simulink model "SSIV_Simulink_Com2"  (R2018a)
settings: Solver=FixedStepAuto  StartTime=0.0  StopTime=inf  FixedStep=.015  RelTol=1e-3  EnableMultiTasking=on
libraries: hdlsllib x51, raspberrypilib x16, simulink x10
(part 2 of 2)

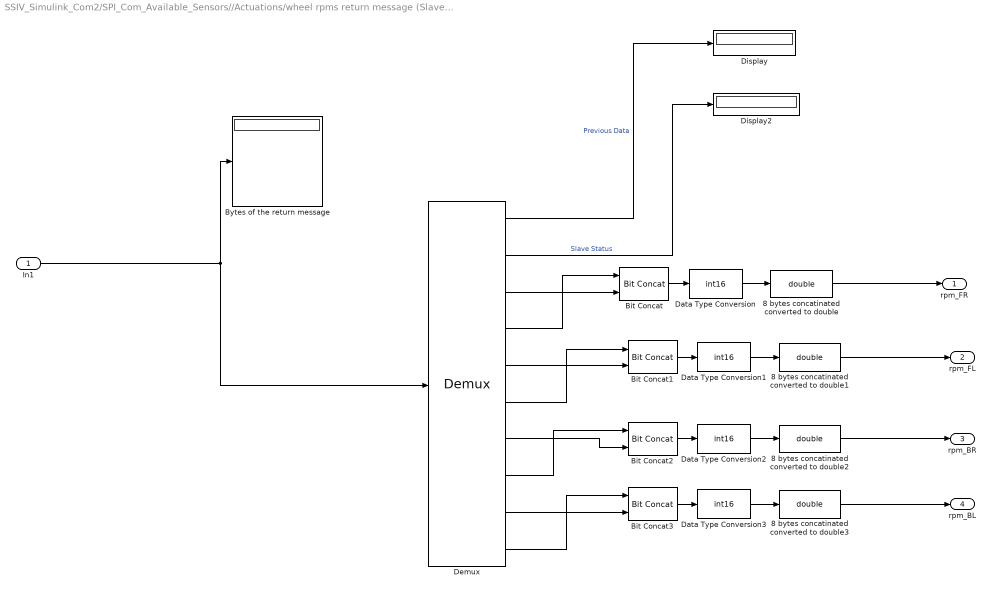
== system SSIV_Simulink_Com2/SPI_Com_Available_Sensors//Actuations/wheel rpms return message (Slave --> Master) ==
  In1 : Inport
  8 bytes concatinated converted to double{,1..3} (4 alike) : DataTypeConversion  OutDataTypeStr=double  RndMeth=Nearest
  Bit Concat{,1..3} (4 alike) : hdlsllib/Logic and Bit Operations/Bit Concat  numInputs=2
      settings: SourceProductName=HDL Coder  SourceProductBaseCode=HD
  Bytes of the return message : Display
      settings: Format=decimal (Stored Integer)
  Data Type Conversion{,1..3} (4 alike) : DataTypeConversion  OutDataTypeStr=int16  RndMeth=Nearest
  Demux : Demux  Outputs=10
  Display : Display
      settings: Format=binary (Stored Integer)
  Display2 : Display
      settings: Format=binary (Stored Integer)
  rpm_FR : Outport
  rpm_FL : Outport  Port=2
  rpm_BR : Outport  Port=3
  rpm_BL : Outport  Port=4
  wires:
  8 bytes concatinated converted to double/1 -> rpm_FR/1
  Demux/2 -> Display2/1  "Slave Status"
  Demux/1 -> Display/1  "Previous Data"
  In1/1 -> Bytes of the return message/1, Demux/1
  Bit Concat/1 -> Data Type Conversion/1
  Demux/4 -> Bit Concat/1
  Demux/3 -> Bit Concat/2
  Data Type Conversion/1 -> 8 bytes concatinated converted to double/1
  Data Type Conversion1/1 -> 8 bytes concatinated converted to double1/1
  Demux/5 -> Bit Concat1/2
  Demux/6 -> Bit Concat1/1
  Bit Concat1/1 -> Data Type Conversion1/1
  8 bytes concatinated converted to double1/1 -> rpm_FL/1
  8 bytes concatinated converted to double2/1 -> rpm_BR/1
  Bit Concat2/1 -> Data Type Conversion2/1
  Demux/8 -> Bit Concat2/1
  Demux/7 -> Bit Concat2/2
  Data Type Conversion2/1 -> 8 bytes concatinated converted to double2/1
  Data Type Conversion3/1 -> 8 bytes concatinated converted to double3/1
  Demux/9 -> Bit Concat3/2
  Demux/10 -> Bit Concat3/1
  Bit Concat3/1 -> Data Type Conversion3/1
  8 bytes concatinated converted to double3/1 -> rpm_BL/1

== system SSIV_Simulink_Com2/SPI_Com_Available_Sensors//Actuations/wheel velocities read message (Master --> Slave) ==
  Inport : Inport
  Mux : Mux  Inputs=10
      settings: DisplayOption=signals
  Read Bit Set : simulink/Logic and Bit Operations/Bit Set  iBit=7
      settings: SourceProductName=Simulink  SourceProductBaseCode=SL
  uint8_t {1..9} (9 alike) : Constant  OutDataTypeStr=uint8
  Out1 : Outport
  wires:
  uint8_t 5/1 -> Mux/6  "Byte 3 will be returned here"
  Mux/1 -> Out1/1
  uint8_t 7/1 -> Mux/8  "Byte 5  will be returned here"
  uint8_t 3/1 -> Mux/4  "Byte 1 will be returned here"
  uint8_t 6/1 -> Mux/7  "Byte 4 will be returned here"
  Read Bit Set/1 -> Mux/1  "Addres/RW Byte rpm front right Teensy Status will be returned here"
  uint8_t 8/1 -> Mux/9  "Byte 6 will be returned here"
  uint8_t 2/1 -> Mux/3  "Byte 0 will be returned here"
  uint8_t 4/1 -> Mux/5  "Byte 2 will be returned here"
  Inport/1 -> Read Bit Set/1
  uint8_t 9/1 -> Mux/10  "Byte 7 will be returned here"
  uint8_t 1/1 -> Mux/2  "Junk will be returned here"

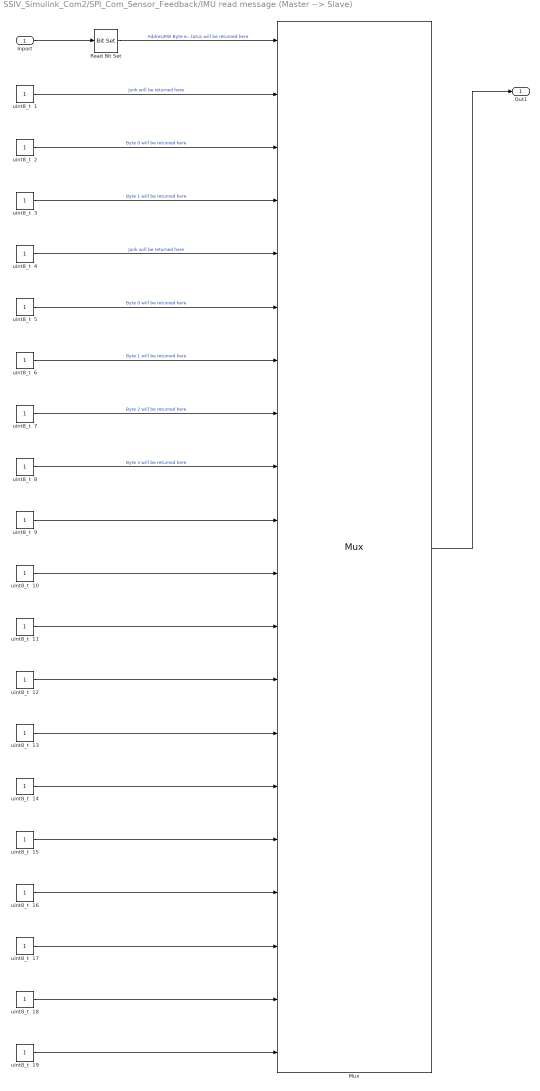
== system SSIV_Simulink_Com2/SPI_Com_Sensor_Feedback/IMU read message (Master --> Slave) ==
  Inport : Inport
  Mux : Mux  Inputs=20
      settings: DisplayOption=signals
  Read Bit Set : simulink/Logic and Bit Operations/Bit Set  iBit=7
      settings: SourceProductName=Simulink  SourceProductBaseCode=SL
  uint8_t  {1..19} (19 alike) : Constant  OutDataTypeStr=uint8
  Out1 : Outport
  wires:
  Read Bit Set/1 -> Mux/1  "Addres/RW Byte euler_heading Teensy Status will be returned here"
  Inport/1 -> Read Bit Set/1
  uint8_t  3/1 -> Mux/4  "Byte 1 will be returned here"
  Mux/1 -> Out1/1
  uint8_t  2/1 -> Mux/3  "Byte 0 will be returned here"
  uint8_t  1/1 -> Mux/2  "Junk will be returned here"
  uint8_t  4/1 -> Mux/5  "Junk will be returned here"
  uint8_t  5/1 -> Mux/6  "Byte 0 will be returned here"
  uint8_t  6/1 -> Mux/7  "Byte 1 will be returned here"
  uint8_t  8/1 -> Mux/9  "Byte 3 will be returned here"
  uint8_t  7/1 -> Mux/8  "Byte 2 will be returned here"
  uint8_t  9/1 -> Mux/10
  uint8_t  16/1 -> Mux/17
  uint8_t  14/1 -> Mux/15
  uint8_t  15/1 -> Mux/16
  uint8_t  13/1 -> Mux/14
  uint8_t  12/1 -> Mux/13
  uint8_t  11/1 -> Mux/12
  uint8_t  10/1 -> Mux/11
  uint8_t  18/1 -> Mux/19
  uint8_t  17/1 -> Mux/18
  uint8_t  19/1 -> Mux/20

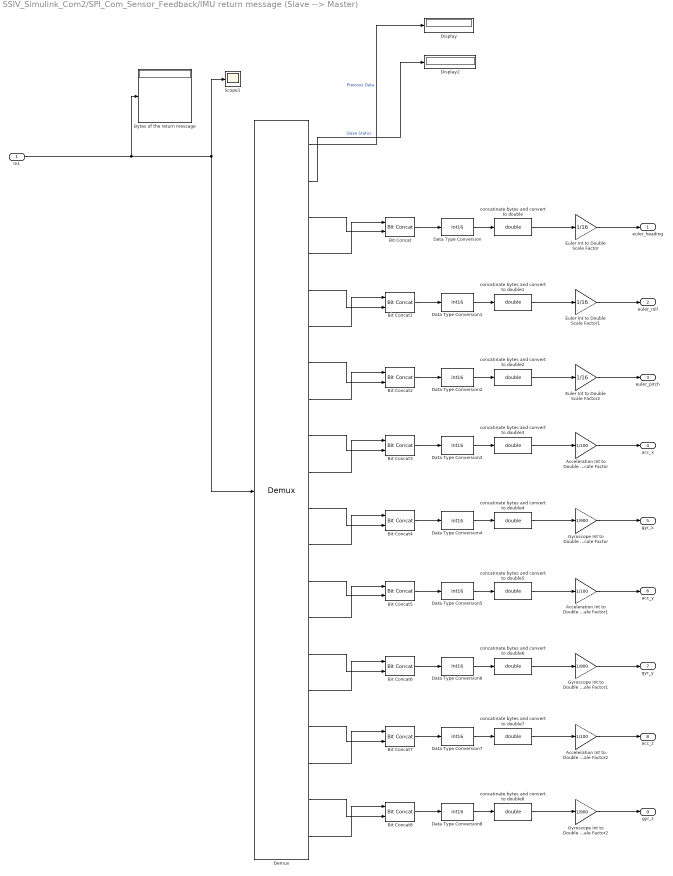
== system SSIV_Simulink_Com2/SPI_Com_Sensor_Feedback/IMU return message (Slave --> Master) ==
  In1 : Inport
  Acceleration Int to Double Scale Factor : Gain  Gain=1/100
  Acceleration Int to Double Scale Factor1 : Gain  Gain=1/100
  Acceleration Int to Double Scale Factor2 : Gain  Gain=1/100
  Bit Concat{,1..8} (9 alike) : hdlsllib/Logic and Bit Operations/Bit Concat  numInputs=2
      settings: SourceProductName=HDL Coder  SourceProductBaseCode=HD
  Bytes of the return message : Display
      settings: Format=decimal (Stored Integer)
  Data Type Conversion{,1..8} (9 alike) : DataTypeConversion  OutDataTypeStr=int16  RndMeth=Nearest
  Demux : Demux  Outputs=20
  Display : Display
      settings: Format=binary (Stored Integer)
  Display2 : Display
      settings: Format=binary (Stored Integer)
  Euler Int to Double Scale Factor : Gain  Gain=1/16
  Euler Int to Double Scale Factor1 : Gain  Gain=1/16
  Euler Int to Double Scale Factor2 : Gain  Gain=1/16
  Gyroscope Int to Double Scale Factor : Gain  Gain=1/900
  Gyroscope Int to Double Scale Factor1 : Gain  Gain=1/900
  Gyroscope Int to Double Scale Factor2 : Gain  Gain=1/900
  Scope1 : Scope
  concatinate bytes and convert to double{,1..8} (9 alike) : DataTypeConversion  OutDataTypeStr=double  RndMeth=Nearest  LockScale=on
  euler_heading : Outport
  euler_roll : Outport  Port=2
  euler_pitch : Outport  Port=3
  acc_x : Outport  Port=4
  gyr_x : Outport  Port=5
  acc_y : Outport  Port=6
  gyr_y : Outport  Port=7
  acc_z : Outport  Port=8
  gyr_z : Outport  Port=9
  wires:
  concatinate bytes and convert to double/1 -> Euler Int to Double Scale Factor/1
  Demux/2 -> Display2/1  "Slave Status"
  Demux/1 -> Display/1  "Previous Data"
  In1/1 -> Bytes of the return message/1, Scope1/1, Demux/1
  Demux/4 -> Bit Concat/1
  Demux/3 -> Bit Concat/2
  Euler Int to Double Scale Factor/1 -> euler_heading/1
  Bit Concat/1 -> Data Type Conversion/1
  Data Type Conversion/1 -> concatinate bytes and convert to double/1
  Data Type Conversion1/1 -> concatinate bytes and convert to double1/1
  Bit Concat1/1 -> Data Type Conversion1/1
  Euler Int to Double Scale Factor1/1 -> euler_roll/1
  Demux/5 -> Bit Concat1/2
  Demux/6 -> Bit Concat1/1
  concatinate bytes and convert to double1/1 -> Euler Int to Double Scale Factor1/1
  concatinate bytes and convert to double2/1 -> Euler Int to Double Scale Factor2/1
  Demux/8 -> Bit Concat2/1
  Demux/7 -> Bit Concat2/2
  Euler Int to Double Scale Factor2/1 -> euler_pitch/1
  Bit Concat2/1 -> Data Type Conversion2/1
  Data Type Conversion2/1 -> concatinate bytes and convert to double2/1
  concatinate bytes and convert to double4/1 -> Gyroscope Int to Double Scale Factor/1
  Demux/12 -> Bit Concat4/1
  Demux/11 -> Bit Concat4/2
  Gyroscope Int to Double Scale Factor/1 -> gyr_x/1
  Bit Concat4/1 -> Data Type Conversion4/1
  Data Type Conversion4/1 -> concatinate bytes and convert to double4/1
  Data Type Conversion3/1 -> concatinate bytes and convert to double3/1
  Bit Concat3/1 -> Data Type Conversion3/1
  Acceleration Int to Double Scale Factor/1 -> acc_x/1
  Demux/9 -> Bit Concat3/2
  Demux/10 -> Bit Concat3/1
  concatinate bytes and convert to double3/1 -> Acceleration Int to Double Scale Factor/1
  concatinate bytes and convert to double5/1 -> Acceleration Int to Double Scale Factor1/1
  Demux/14 -> Bit Concat5/1
  Demux/13 -> Bit Concat5/2
  Acceleration Int to Double Scale Factor1/1 -> acc_y/1
  Bit Concat5/1 -> Data Type Conversion5/1
  Data Type Conversion5/1 -> concatinate bytes and convert to double5/1
  Data Type Conversion6/1 -> concatinate bytes and convert to double6/1
  Bit Concat6/1 -> Data Type Conversion6/1
  Gyroscope Int to Double Scale Factor1/1 -> gyr_y/1
  Demux/15 -> Bit Concat6/2
  Demux/16 -> Bit Concat6/1
  concatinate bytes and convert to double6/1 -> Gyroscope Int to Double Scale Factor1/1
  concatinate bytes and convert to double8/1 -> Gyroscope Int to Double Scale Factor2/1
  Demux/20 -> Bit Concat8/1
  Demux/19 -> Bit Concat8/2
  Gyroscope Int to Double Scale Factor2/1 -> gyr_z/1
  Bit Concat8/1 -> Data Type Conversion8/1
  Data Type Conversion8/1 -> concatinate bytes and convert to double8/1
  Data Type Conversion7/1 -> concatinate bytes and convert to double7/1
  Bit Concat7/1 -> Data Type Conversion7/1
  Acceleration Int to Double Scale Factor2/1 -> acc_z/1
  Demux/17 -> Bit Concat7/2
  Demux/18 -> Bit Concat7/1
  concatinate bytes and convert to double7/1 -> Acceleration Int to Double Scale Factor2/1

== system SSIV_Simulink_Com2/SPI_Com_Sensor_Feedback/radio throttle and steering read message (Master --> Slave) ==
  Inport : Inport
  Mux : Mux  Inputs=6
      settings: DisplayOption=signals
  Read Bit Set : simulink/Logic and Bit Operations/Bit Set  iBit=7
      settings: SourceProductName=Simulink  SourceProductBaseCode=SL
  uint8_t {1..5} (5 alike) : Constant  OutDataTypeStr=uint8
  Out1 : Outport
  wires:
  Read Bit Set/1 -> Mux/1  "Addres/RW Byte radio_throttle Teensy Status will be returned here"
  uint8_t 1/1 -> Mux/2  "Junk will be returned here"
  Inport/1 -> Read Bit Set/1
  uint8_t 3/1 -> Mux/4  "Byte 1 will be returned here"
  Mux/1 -> Out1/1
  uint8_t 2/1 -> Mux/3  "Byte 0 will be returned here"
  uint8_t 4/1 -> Mux/5  "Byte 2 will be returned here"
  uint8_t 5/1 -> Mux/6  "Byte 3 will be returned here"

== system SSIV_Simulink_Com2/SPI_Com_Sensor_Feedback/radio throttle and steering return message (Slave --> Master) ==
  In1 : Inport
  8 bytes concatinated converted to double : DataTypeConversion  OutDataTypeStr=double  RndMeth=Nearest
  8 bytes concatinated converted to double1 : DataTypeConversion  OutDataTypeStr=double  RndMeth=Nearest
  Bit Concat : hdlsllib/Logic and Bit Operations/Bit Concat  numInputs=2
      settings: SourceProductName=HDL Coder  SourceProductBaseCode=HD
  Bit Concat1 : hdlsllib/Logic and Bit Operations/Bit Concat  numInputs=2
      settings: SourceProductName=HDL Coder  SourceProductBaseCode=HD
  Bytes of the return message : Display
      settings: Format=decimal (Stored Integer)
  Data Type Conversion : DataTypeConversion  OutDataTypeStr=int16  RndMeth=Nearest
  Data Type Conversion1 : DataTypeConversion  OutDataTypeStr=int16  RndMeth=Nearest
  Demux : Demux  Outputs=6
  Display : Display
      settings: Format=binary (Stored Integer)
  Display2 : Display
      settings: Format=binary (Stored Integer)
  radio_throttle : Outport
  radio_steering : Outport  Port=2
  wires:
  8 bytes concatinated converted to double/1 -> radio_throttle/1
  Demux/2 -> Display2/1  "Slave Status"
  Demux/1 -> Display/1  "Previous Data"
  In1/1 -> Bytes of the return message/1, Demux/1
  Bit Concat/1 -> Data Type Conversion/1
  Demux/4 -> Bit Concat/1
  Demux/3 -> Bit Concat/2
  Data Type Conversion/1 -> 8 bytes concatinated converted to double/1
  Data Type Conversion1/1 -> 8 bytes concatinated converted to double1/1
  Demux/5 -> Bit Concat1/2
  Demux/6 -> Bit Concat1/1
  Bit Concat1/1 -> Data Type Conversion1/1
  8 bytes concatinated converted to double1/1 -> radio_steering/1

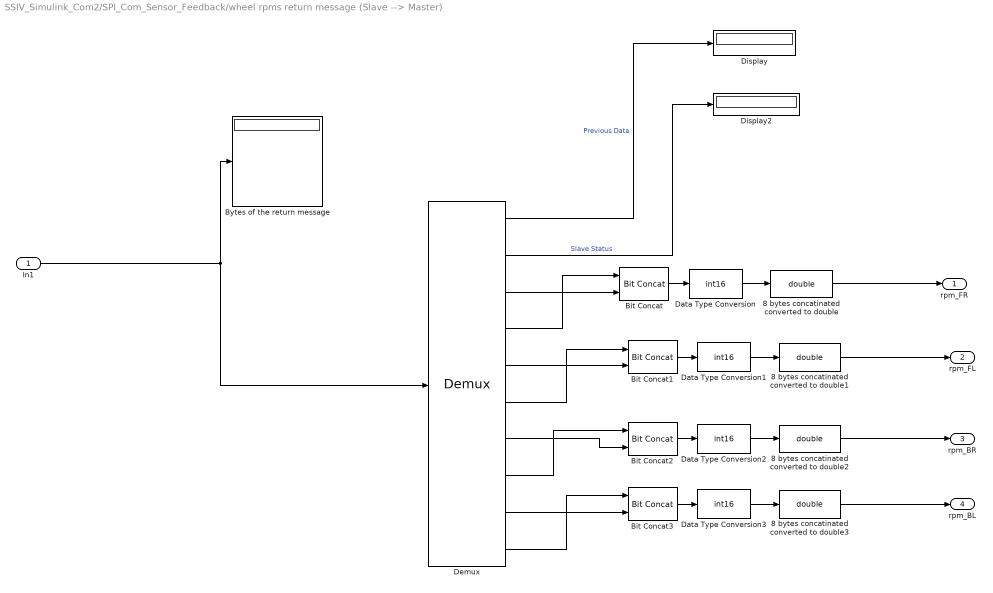
== system SSIV_Simulink_Com2/SPI_Com_Sensor_Feedback/wheel rpms return message (Slave --> Master) ==
  In1 : Inport
  8 bytes concatinated converted to double{,1..3} (4 alike) : DataTypeConversion  OutDataTypeStr=double  RndMeth=Nearest
  Bit Concat{,1..3} (4 alike) : hdlsllib/Logic and Bit Operations/Bit Concat  numInputs=2
      settings: SourceProductName=HDL Coder  SourceProductBaseCode=HD
  Bytes of the return message : Display
      settings: Format=decimal (Stored Integer)
  Data Type Conversion{,1..3} (4 alike) : DataTypeConversion  OutDataTypeStr=int16  RndMeth=Nearest
  Demux : Demux  Outputs=10
  Display : Display
      settings: Format=binary (Stored Integer)
  Display2 : Display
      settings: Format=binary (Stored Integer)
  rpm_FR : Outport
  rpm_FL : Outport  Port=2
  rpm_BR : Outport  Port=3
  rpm_BL : Outport  Port=4
  wires:
  8 bytes concatinated converted to double/1 -> rpm_FR/1
  Demux/2 -> Display2/1  "Slave Status"
  Demux/1 -> Display/1  "Previous Data"
  In1/1 -> Bytes of the return message/1, Demux/1
  Bit Concat/1 -> Data Type Conversion/1
  Demux/4 -> Bit Concat/1
  Demux/3 -> Bit Concat/2
  Data Type Conversion/1 -> 8 bytes concatinated converted to double/1
  Data Type Conversion1/1 -> 8 bytes concatinated converted to double1/1
  Demux/5 -> Bit Concat1/2
  Demux/6 -> Bit Concat1/1
  Bit Concat1/1 -> Data Type Conversion1/1
  8 bytes concatinated converted to double1/1 -> rpm_FL/1
  8 bytes concatinated converted to double2/1 -> rpm_BR/1
  Bit Concat2/1 -> Data Type Conversion2/1
  Demux/8 -> Bit Concat2/1
  Demux/7 -> Bit Concat2/2
  Data Type Conversion2/1 -> 8 bytes concatinated converted to double2/1
  Data Type Conversion3/1 -> 8 bytes concatinated converted to double3/1
  Demux/9 -> Bit Concat3/2
  Demux/10 -> Bit Concat3/1
  Bit Concat3/1 -> Data Type Conversion3/1
  8 bytes concatinated converted to double3/1 -> rpm_BL/1

== system SSIV_Simulink_Com2/SPI_Com_Sensor_Feedback/wheel velocities read message (Master --> Slave) ==
  Inport : Inport
  Mux : Mux  Inputs=10
      settings: DisplayOption=signals
  Read Bit Set : simulink/Logic and Bit Operations/Bit Set  iBit=7
      settings: SourceProductName=Simulink  SourceProductBaseCode=SL
  uint8_t {1..9} (9 alike) : Constant  OutDataTypeStr=uint8
  Out1 : Outport
  wires:
  uint8_t 5/1 -> Mux/6  "Byte 3 will be returned here"
  Mux/1 -> Out1/1
  uint8_t 7/1 -> Mux/8  "Byte 5  will be returned here"
  uint8_t 3/1 -> Mux/4  "Byte 1 will be returned here"
  uint8_t 6/1 -> Mux/7  "Byte 4 will be returned here"
  Read Bit Set/1 -> Mux/1  "Addres/RW Byte rpm front right Teensy Status will be returned here"
  uint8_t 8/1 -> Mux/9  "Byte 6 will be returned here"
  uint8_t 2/1 -> Mux/3  "Byte 0 will be returned here"
  uint8_t 4/1 -> Mux/5  "Byte 2 will be returned here"
  Inport/1 -> Read Bit Set/1
  uint8_t 9/1 -> Mux/10  "Byte 7 will be returned here"
  uint8_t 1/1 -> Mux/2  "Junk will be returned here"

== system SSIV_Simulink_Com2/SPI_Com_Servo_Out/servo_out Write Message (Master --> Slave) ==
  In1 : Inport
  Bit Slice2 : hdlsllib/Logic and Bit Operations/Bit Slice  lidx=15  ridx=8
  Bit Slice3 : hdlsllib/Logic and Bit Operations/Bit Slice  lidx=7  ridx=0
  Display5 : Display
      settings: Format=decimal (Stored Integer)
  Mux : Mux  Inputs=2
      settings: DisplayOption=signals
  Out1 : Outport
  wires:
  In1/1 -> Display5/1, Bit Slice3/1, Bit Slice2/1  "Servo"
  Mux/1 -> Out1/1
  Bit Slice3/1 -> Mux/1
  Bit Slice2/1 -> Mux/2

== system SSIV_Simulink_Com2/Controller_Example/SPI_Communication_Torque_Actuations/torque Write Message (Master --> Slave) ==
  In1 : Inport
  In2 : Inport  Port=2
  In3 : Inport  Port=3
  In4 : Inport  Port=4
  Bit Slice{,2,4,6} (4 alike) : hdlsllib/Logic and Bit Operations/Bit Slice  lidx=15  ridx=8
  Bit Slice{1,3,5,7} (4 alike) : hdlsllib/Logic and Bit Operations/Bit Slice  lidx=7  ridx=0
  Mux : Mux  Inputs=8
      settings: DisplayOption=signals
  Output : Outport
  wires:
  Bit Slice/1 -> Mux/2
  Bit Slice1/1 -> Mux/1
  In1/1 -> Bit Slice/1, Bit Slice1/1
  In2/1 -> Bit Slice3/1, Bit Slice2/1
  Bit Slice3/1 -> Mux/3
  Bit Slice2/1 -> Mux/4
  Bit Slice4/1 -> Mux/6
  Bit Slice5/1 -> Mux/5
  In3/1 -> Bit Slice4/1, Bit Slice5/1
  In4/1 -> Bit Slice7/1, Bit Slice6/1
  Bit Slice7/1 -> Mux/7
  Bit Slice6/1 -> Mux/8
  Mux/1 -> Output/1
